simulink model "TBCC_Dyn"  (Simulink 10.0)
settings: Solver=VariableStepAuto  StartTime=0.0  StopTime=MWS.in.SimTime  FixedStep=MWS.Solve.T  RelTol=1e-3
values from neighbouring files (symbols this model uses):
  MWS = setup_Inlet(MWS)    [TBCC_setup_everything.m]
undefined symbols (not defined in the file or in its folder): combustion, diffuser, g, gama_ho, inlet_v, L_ho, nozzle, Pa, Pc_ho, R, R_ho, r_ho, stripchar_TMATS, Tc_ho, Wt_ho
libraries: Lib_Solve_ModelSource_TMATS x10, simulink_extras x7, Lib_Cntrl_FirstOrderSensor_TMATS x2, Lib_Solve_OuterLoopIntegrator_TMATS x2, Lib_Cntrl_SimplePIcontroller_TMATS x2, Lib_Turbo_Ambient_TMATS x2, Lib_Turbo_Burner_TMATS x2, Lib_Turbo_Compressor_TMATS x2, Lib_Turbo_Duct_TMATS x2, Lib_Turbo_Inlet_TMATS x2, Lib_Turbo_Nozzle_TMATS x2, Lib_Turbo_Shaft_TMATS x2
(part 1 of 2)
CloseFcn:
  | run(strcat(MWS.top_level, filesep,'GasTurbine_Dyn_Example_cleanup'))
settings Model: Creator=jwchapm2  LastModifiedBy=114-AO  SimulationMode=accelerator
settings SolverCC: AutoInsertRateTranBlk=on
settings DataIOCC: LimitDataPoints=on  SignalLoggingName=SimulationOutput
settings OptimizationCC: BlockReduction=off  DefaultParameterBehavior=Inlined  BufferReuse=off  ExpressionDepthLimit=2147483647
settings DebuggingCC: SolverPrmCheckMsg=warning  MultiTaskCondExecSysMsg=none  StateNameClashWarn=warning
settings GRTTargetCC: GeneratePreprocessorConditionals=Disable all  CombineOutputUpdateFcns=on  GRTInterface=off
settings ConfigComp: CovExternalEMLEnable=off

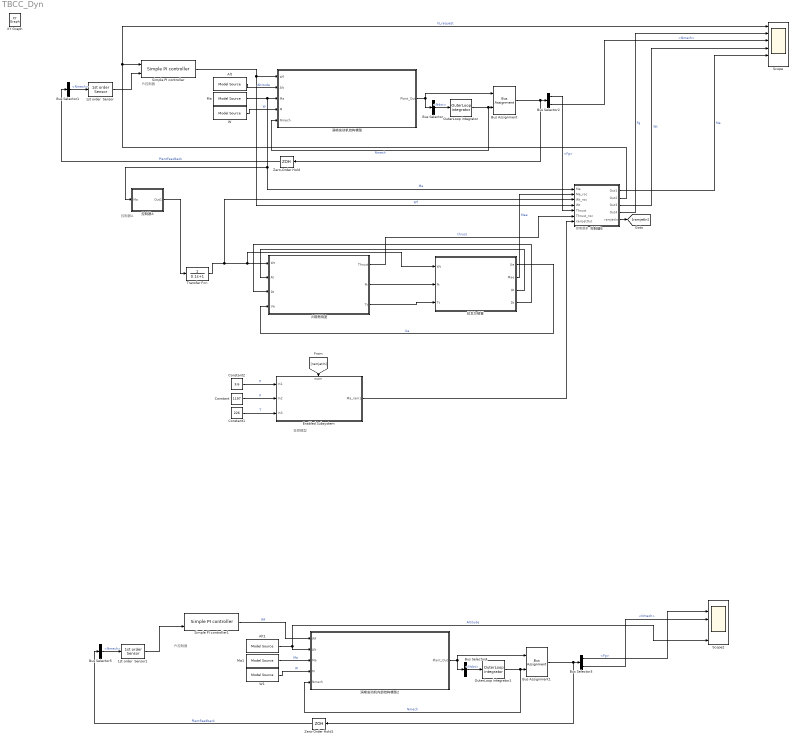
== system TBCC_Dyn ==
  note: 亚燃模型
  note: PI控制器
  note: 控制器A
  note: 控制器B
  note: PI控制器
  1st order  Sensor : Lib_Cntrl_FirstOrderSensor_TMATS/1st order  Sensor  IC_M=MWS.Solve.N_IC  Sen_Max_M=20000  Sen_Min_M=0  Gain_M=1  Tau_M=0.05  GN_EN_M=off  GN_NST_M=MWS.Solve.T  GN_C_M=1  GN_MinNoise_M=0.3  F_Gain_M=1  F_Drift_M=0
  1st order  Sensor1 : Lib_Cntrl_FirstOrderSensor_TMATS/1st order  Sensor  IC_M=MWS.Solve.N_IC  Sen_Max_M=20000  Sen_Min_M=0  Gain_M=1  Tau_M=0.05  GN_EN_M=off  GN_NST_M=MWS.Solve.T  GN_C_M=1  GN_MinNoise_M=0.3  F_Gain_M=1  F_Drift_M=0
  Alt : Lib_Solve_ModelSource_TMATS/Model Source  T_vec_M=MWS.in.t_vec  input_array_M=MWS.in.Alt
  Alt1 : Lib_Solve_ModelSource_TMATS/Model Source  T_vec_M=MWS.in.t_vec  input_array_M=MWS.in.Alt
  Bus Assignment : BusAssignment  AssignedSignals=PlantBus.Nmech
  Bus Assignment1 : BusAssignment  AssignedSignals=PlantBus.Nmech
  Bus Selector2 : BusSelector  OutputSignals=PlantBus.Fg,PlantBus.Nmech
  Bus Selector3 : BusSelector  OutputSignals=PlantBus.Fg,PlantBus.Nmech
  Bus Selector : BusSelector  OutputSignals=PlantBus.Ndot
  Bus Selector1 : BusSelector  OutputSignals=PlantBus.Nmech
  Bus Selector4 : BusSelector  OutputSignals=PlantBus.Ndot
  Bus Selector5 : BusSelector  OutputSignals=PlantBus.Nmech
  Constant : Constant  Value=1197
  Constant1 : Constant  Value=226
  Constant2 : Constant  Value=3.6
  Enabled Subsystem : Subsystem  TreatAsAtomicUnit=on
      mask Display: image('ramjet.jpg'); % Use "Edit Image" on toolstrip to change.
  Ma : Lib_Solve_ModelSource_TMATS/Model Source  T_vec_M=MWS.in.t_vec  input_array_M=MWS.in.Ma
  Ma1 : Lib_Solve_ModelSource_TMATS/Model Source  T_vec_M=MWS.in.t_vec  input_array_M=MWS.in.Ma
  OuterLoop integrator : Lib_Solve_OuterLoopIntegrator_TMATS/OuterLoop integrator  OL_IC_M=MWS.Solve.N_IC
  OuterLoop integrator1 : Lib_Solve_OuterLoopIntegrator_TMATS/OuterLoop integrator  OL_IC_M=MWS.Solve.N_IC
  Scope : Scope  NumInputPorts=6
  Scope2 : Scope  NumInputPorts=6
  Simple PI controller : Lib_Cntrl_SimplePIcontroller_TMATS/Simple PI controller  Kp_M=0.05/2  Ki_M=0.1/2  PI_IC_M=3
  Simple PI controller1 : Lib_Cntrl_SimplePIcontroller_TMATS/Simple PI controller  Kp_M=0.05/2  Ki_M=0.1/2  PI_IC_M=3
  Transfer Fcn : TransferFcn  Denominator=[0.1 1]
  W : Lib_Solve_ModelSource_TMATS/Model Source  T_vec_M=MWS.in.t_vec  input_array_M=MWS.in.W
  W1 : Lib_Solve_ModelSource_TMATS/Model Source  T_vec_M=MWS.in.t_vec  input_array_M=MWS.in.W
  Zero-Order Hold : ZeroOrderHold  SampleTime=MWS.Solve.T
  Zero-Order Hold1 : ZeroOrderHold  SampleTime=MWS.Solve.T
  拉瓦尔喷管 : Subsystem
      mask Display: image('lawaer.jpg'); % Use "Edit Image" on toolstrip to change.
  控制器A : Subsystem
  控制器B : Subsystem
  涡喷发动机内部结构模型2 : Subsystem
      mask Display: image('turbine.jpg'); % Use "Edit Image" on toolstrip to change.
  涡喷发动机结构模型 : Subsystem
      mask Display: image('turbine.jpg'); % Use "Edit Image" on toolstrip to change.
  火箭燃烧室 : Subsystem
      mask Display: image('rocket.jpg'); % Use "Edit Image" on toolstrip to change.
  XY Graph : simulink/Sinks/XY Graph  IOType=viewer  xmin=-1  xmax=1  ymin=-1  ymax=1  st=-1
  wires:
  Zero-Order Hold/1 -> Bus Selector1/1  "PlantFeedback"
  涡喷发动机结构模型/1(Plant_Out) -> Bus Selector/1, Bus Assignment/1
  Bus Selector/1 -> OuterLoop integrator/1  "<Ndot>"
  Bus Assignment/1 -> Bus Selector2/1, Zero-Order Hold/1
  OuterLoop integrator/1 -> 涡喷发动机结构模型/5(Nmech), Bus Assignment/2  "Nmech"
  Bus Selector1/1 -> 1st order  Sensor/1  "<Nmech>"
  Simple PI controller/1 -> 涡喷发动机结构模型/1(Wf), 控制器B/4(Wt)  "Wf"
  1st order  Sensor/1 -> Simple PI controller/2
  Alt/1 -> 涡喷发动机结构模型/2(Alt)  "Altitude"
  Ma/1 -> 控制器B/1(Ma), 控制器A/1(Ma), 涡喷发动机结构模型/3(Ma)  "Ma"
  W/1 -> 涡喷发动机结构模型/4(M)  "W"
  Bus Selector2/2 -> Scope/3  "<Nmech>"
  拉瓦尔喷管/4(Dt) -> 火箭燃烧室/3(Dt)
  Transfer Fcn/1 -> 控制器B/3(Wt_roc), 拉瓦尔喷管/1(Wt), 火箭燃烧室/1(Wt)
  火箭燃烧室/2(Pt) -> 拉瓦尔喷管/2(Pt)
  拉瓦尔喷管/1(Ue) -> 火箭燃烧室/4(Ue)  "Ue"
  拉瓦尔喷管/3(At) -> 火箭燃烧室/2(At)
  火箭燃烧室/3(Tt) -> 拉瓦尔喷管/3(Tt)
  拉瓦尔喷管/2(Mae) -> 控制器B/2(Ma_roc)  "Mae"
  控制器B/1(Out1) -> Scope/5  "Ma"
  控制器A/1(Out1) -> Transfer Fcn/1
  控制器B/3(Out3) -> Scope/4  "Wt"
  Bus Selector2/1 -> 控制器B/5(Thrust)  "<Fg>"
  火箭燃烧室/1(Thrust) -> 控制器B/6(Thrust_roc)  "thrust"
  控制器B/4(Out4) -> Scope/2  "Fg"
  Alt1/1 -> Scope2/6, 涡喷发动机内部结构模型2/2(Alt)  "Altitude"
  Bus Selector3/2 -> Scope2/3  "<Nmech>"
  W1/1 -> 涡喷发动机内部结构模型2/4(M)  "W"
  Ma1/1 -> 涡喷发动机内部结构模型2/3(Ma)  "Ma"
  控制器B/2(Out2) -> Simple PI controller/1, Scope/1  "N_request"
  涡喷发动机内部结构模型2/1(Plant_Out) -> Bus Selector4/1, Bus Assignment1/1
  1st order  Sensor1/1 -> Simple PI controller1/2
  Simple PI controller1/1 -> 涡喷发动机内部结构模型2/1(Wf)  "Wf"
  OuterLoop integrator1/1 -> 涡喷发动机内部结构模型2/5(Nmech), Bus Assignment1/2  "Nmech"
  Zero-Order Hold1/1 -> Bus Selector5/1  "PlantFeedback"
  Bus Assignment1/1 -> Bus Selector3/1, Zero-Order Hold1/1
  Bus Selector5/1 -> 1st order  Sensor1/1  "<Nmech>"
  Bus Selector4/1 -> OuterLoop integrator1/1  "<Ndot>"
  Bus Selector3/1 -> Scope2/2  "<Fg>"
  控制器B/5(ramjetIn) -> [ramjetIn]
  [ramjetIn] -> Enabled Subsystem/Enable
  Constant2/1 -> Enabled Subsystem/1(In1)  "P"
  Constant/1 -> Enabled Subsystem/2(In2)  "P"
  Constant1/1 -> Enabled Subsystem/3(In3)  "T"
  Enabled Subsystem/1(Ma_ram1) -> 控制器B/7(ramjetOut)

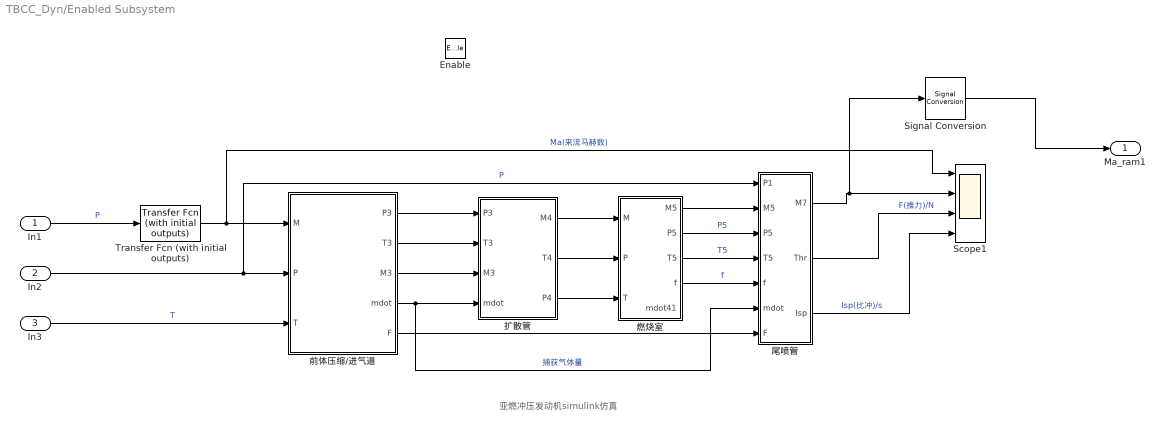
== system TBCC_Dyn/Enabled Subsystem ==
  note: 亚燃冲压发动机simulink仿真
  In1 : Inport
  In2 : Inport  Port=2
  In3 : Inport  Port=3
  Enable : EnablePort
  Scope1 : Scope  NumInputPorts=4
  Signal Conversion : SignalConversion  OverrideOpt=off
  Transfer Fcn (with initial outputs) : simulink_extras/Additional Linear/Transfer Fcn (with initial outputs)  N=[1]  D="[2  1]"  Y0=2.6  U0=0
  前体压缩/进气道 : Subsystem
  尾喷管 : Subsystem
  扩散管 : Subsystem
  燃烧室 : Subsystem
  Ma_ram1 : Outport
  wires:
  Signal Conversion/1 -> Ma_ram1/1
  扩散管/1(M4) -> 燃烧室/1(M)
  扩散管/3(P4) -> 燃烧室/3(T)
  In1/1 -> Transfer Fcn (with initial outputs)/1  "P"
  前体压缩/进气道/3(M3) -> 扩散管/3(M3)
  前体压缩/进气道/5(F) -> 尾喷管/7(F)
  前体压缩/进气道/1(P3) -> 扩散管/1(P3)
  尾喷管/1(M7) -> Signal Conversion/1, Scope1/2
  燃烧室/1(M5) -> 尾喷管/2(M5)
  In3/1 -> 前体压缩/进气道/3(T)  "T"
  燃烧室/3(T5) -> 尾喷管/4(T5)  "T5"
  In2/1 -> 尾喷管/1(P1), 前体压缩/进气道/2(P)  "P"
  Transfer Fcn (with initial outputs)/1 -> Scope1/1, 前体压缩/进气道/1(M)  "Ma(来流马赫数)"
  燃烧室/2(P5) -> 尾喷管/3(P5)  "P5"
  前体压缩/进气道/2(T3) -> 扩散管/2(T3)
  前体压缩/进气道/4(mdot) -> 尾喷管/6(mdot), 扩散管/4(mdot)  "捕获气体量"
  扩散管/2(T4) -> 燃烧室/2(P)
  尾喷管/3(Isp) -> Scope1/4  "Isp(比冲)/s"
  燃烧室/4(f) -> 尾喷管/5(f)  "f"
  尾喷管/2(Thr) -> Scope1/3  "F(推力)/N"

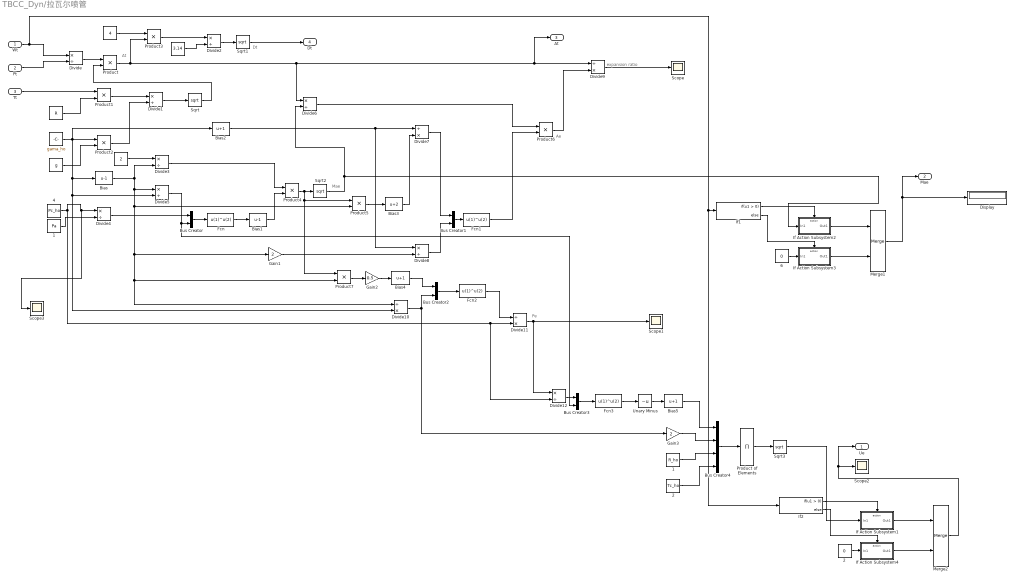
== system TBCC_Dyn/拉瓦尔喷管 ==
  note: expansion ratio
  note: Dt
  note: At
  note: Mae
  note: Ae
  note: Pe
  Wt : Inport
  Pt : Inport  Port=2
  Tt : Inport  Port=3
  " " : Constant  Value=R  SampleTime=0.6
  "  " : Constant  Value=gama_ho  SampleTime=0.6
  "   " : Constant  Value=4  SampleTime=0.6
  "    " : Constant  Value=g  SampleTime=0.6
  "     " : Constant  Value=3.14  SampleTime=0.6
  "        " : Constant  Value=2  SampleTime=0.6
  "    1" : Constant  Value=Pa  SampleTime=0.6
  "    2" : Constant  Value=0  SampleTime=0.6
  "    4" : Constant  Value=Pc_ho  SampleTime=0.6
  "    6" : Constant  Value=0  SampleTime=0.6
  " 1" : Constant  Value=R_ho  SampleTime=0.6
  " 2" : Constant  Value=Tc_ho  SampleTime=0.6
  Bias : Bias  Bias=-1
  Bias1 : Bias  Bias=-1
  Bias2 : Bias  Bias=1
  Bias3 : Bias  Bias=2
  Bias4 : Bias  Bias=1
  Bias5 : Bias  Bias=1
  Bus Creator{,1..3} (4 alike) : BusCreator  Inputs=2
  Bus Creator4 : BusCreator  Inputs=4
  Display : Display
  Divide{,1..6,8,12} (9 alike) : Product  Inputs=*/
  Divide{7,9..11} (4 alike) : Product  Inputs=/*
  Fcn{,1..3} (4 alike) : Fcn  Expr=u(1)^u(2)
  Gain1 : Gain  Gain=2
  Gain2 : Gain  Gain=0.5
  Gain3 : Gain  Gain=2
  If Action Subsystem1 : Subsystem  TreatAsAtomicUnit=on
  If Action Subsystem2 : Subsystem  TreatAsAtomicUnit=on
  If Action Subsystem3 : Subsystem  TreatAsAtomicUnit=on
  If Action Subsystem4 : Subsystem  TreatAsAtomicUnit=on
  If1 : If
  If2 : If
  Merge1 : Merge
  Merge2 : Merge
  Product{,1..7} (8 alike) : Product
  Product of Elements : Product  Inputs=*
  Scope{,1..3} (4 alike) : Scope
  Sqrt{,1..3} (4 alike) : Sqrt  SaturateOnIntegerOverflow=on
  Unary Minus : UnaryMinus
  Ue : Outport
  Mae : Outport  Port=2
  At : Outport  Port=3
  Dt : Outport  Port=4
  wires:
  Pt/1 -> Divide/2
  Divide/1 -> Product/1
  Tt/1 -> Product1/1
  " "/1 -> Product1/2
  Product1/1 -> Divide1/1
  "  "/1 -> Bias2/1, Divide10/2, Divide5/2, Bias/1, Product2/1
  "    "/1 -> Product2/2
  Product2/1 -> Divide1/2
  Divide1/1 -> Sqrt/1
  Sqrt/1 -> Product/2
  Product/1 -> Product3/2, Divide6/1, At/1, Divide9/1
  "   "/1 -> Product3/1
  Product3/1 -> Divide2/1
  "     "/1 -> Divide2/2
  Divide2/1 -> Sqrt1/1
  Sqrt1/1 -> Dt/1
  Bias/1 -> Divide10/1, Product7/2, Gain1/1, Product5/2, Divide5/1, Divide3/2
  "        "/1 -> Divide3/1
  "    1"/1 -> Divide4/2
  Divide5/1 -> Bus Creator3/2, Bus Creator/2
  Divide4/1 -> Bus Creator/1
  Bus Creator/1 -> Fcn/1
  Fcn/1 -> Bias1/1
  Divide3/1 -> Product4/1
  Bias1/1 -> Product4/2
  Product4/1 -> Product7/1, Product5/1, Sqrt2/1
  Product5/1 -> Bias3/1
  Bias3/1 -> Divide7/2
  Bias2/1 -> Divide7/1, Divide8/1
  Gain1/1 -> Divide8/2
  Divide7/1 -> Bus Creator1/1
  Divide8/1 -> Bus Creator1/2
  Bus Creator1/1 -> Fcn1/1
  Divide6/1 -> Product6/1
  Fcn1/1 -> Product6/2
  Product6/1 -> Divide9/2
  Divide9/1 -> Scope/1
  Product7/1 -> Gain2/1
  Gain2/1 -> Bias4/1
  Bias4/1 -> Bus Creator2/1
  Divide10/1 -> Gain3/1, Bus Creator2/2
  Bus Creator2/1 -> Fcn2/1
  Fcn2/1 -> Divide11/1
  Divide11/1 -> Divide12/1, Scope1/1
  Bus Creator3/1 -> Fcn3/1
  Divide12/1 -> Bus Creator3/1
  Fcn3/1 -> Unary Minus/1
  Unary Minus/1 -> Bias5/1
  Gain3/1 -> Bus Creator4/2
  " 1"/1 -> Bus Creator4/3
  " 2"/1 -> Bus Creator4/4
  Product of Elements/1 -> Sqrt3/1
  Bias5/1 -> Bus Creator4/1
  Bus Creator4/1 -> Product of Elements/1
  Merge2/1 -> Ue/1, Scope2/1
  Wt/1 -> If2/1, If1/1, Divide/1
  "    4"/1 -> Divide12/2, Divide11/2, Scope3/1, Divide4/1
  If1/2 -> If Action Subsystem3/Action
  Sqrt2/1 -> If Action Subsystem2/1(In1), Divide6/2
  "    6"/1 -> If Action Subsystem3/1(In1)
  If Action Subsystem3/1(Out1) -> Merge1/2
  If1/1 -> If Action Subsystem2/Action
  Merge1/1 -> Display/1, Mae/1
  If Action Subsystem2/1(Out1) -> Merge1/1
  If2/2 -> If Action Subsystem4/Action
  If2/1 -> If Action Subsystem1/Action
  "    2"/1 -> If Action Subsystem4/1(In1)
  If Action Subsystem4/1(Out1) -> Merge2/2
  If Action Subsystem1/1(Out1) -> Merge2/1
  Sqrt3/1 -> If Action Subsystem1/1(In1)

== system TBCC_Dyn/控制器A ==
  Ma : Inport
  "    3" : Constant  Value=0  SampleTime=0.6
  If : If  IfExpression=u1 >= 1
  If Action Subsystem : Subsystem  TreatAsAtomicUnit=on
  If Action Subsystem1 : Subsystem  TreatAsAtomicUnit=on
  Merge : Merge
  Wt : Constant  Value=Wt_ho  SampleTime=0.6
  Out1 : Outport
  wires:
  Merge/1 -> Out1/1
  "    3"/1 -> If Action Subsystem1/1(In1)
  Wt/1 -> If Action Subsystem/1(In1)
  If/2 -> If Action Subsystem1/Action
  If Action Subsystem/1(Out1) -> Merge/1
  If/1 -> If Action Subsystem/Action
  If Action Subsystem1/1(Out1) -> Merge/2
  Ma/1 -> If/1

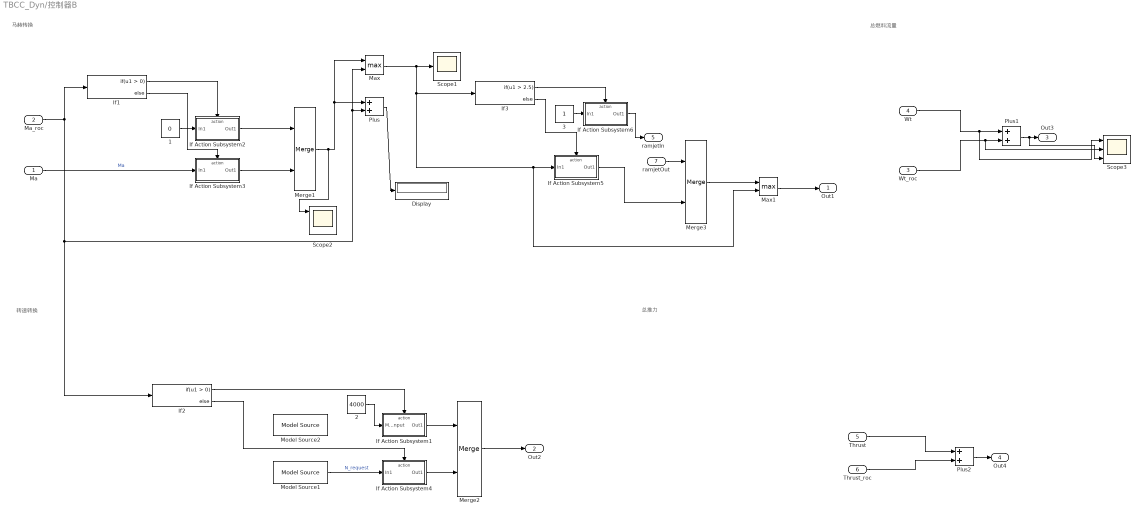
== system TBCC_Dyn/控制器B ==
  note: 总燃料流量
  note: 马赫转换
  note: 转速转换
  note: 总推力
  Ma : Inport
  Ma_roc : Inport  Port=2
  Wt_roc : Inport  Port=3
  Wt : Inport  Port=4
  Thrust : Inport  Port=5
  Thrust_roc : Inport  Port=6
  ramjetOut : Inport  Port=7
  "    1" : Constant  Value=0  SampleTime=0.6
  "    2" : Constant  Value=4000  SampleTime=0.6
  "    3" : Constant  SampleTime=0.6
  Display : Display
  If Action Subsystem1 : Subsystem  TreatAsAtomicUnit=on
  If Action Subsystem2 : Subsystem  TreatAsAtomicUnit=on
  If Action Subsystem3 : Subsystem  TreatAsAtomicUnit=on
  If Action Subsystem4 : Subsystem  TreatAsAtomicUnit=on
  If Action Subsystem5 : Subsystem  TreatAsAtomicUnit=on
  If Action Subsystem6 : Subsystem  TreatAsAtomicUnit=on
  If1 : If
  If2 : If
  If3 : If  IfExpression=u1 > 2.5
  Max : MinMax  Function=max  Inputs=2
  Max1 : MinMax  Function=max  Inputs=2
  Merge1 : Merge  InitialOutput=[1]
  Merge2 : Merge  InitialOutput=[1]
  Merge3 : Merge  InitialOutput=[1]
  Model Source1 : Lib_Solve_ModelSource_TMATS/Model Source  T_vec_M=MWS.in.t_vec  input_array_M=MWS.in.Ndmd
  Model Source2 : Lib_Solve_ModelSource_TMATS/Model Source  T_vec_M=MWS.in.t_vec  input_array_M=MWS.in.Ndmd_stop
  Plus : Sum
  Plus1 : Sum
  Plus2 : Sum
  Scope1 : Scope  NumInputPorts=3
  Scope2 : Scope  NumInputPorts=3
  Scope3 : Scope  NumInputPorts=3
  Out1 : Outport
  Out2 : Outport  Port=2
  Out3 : Outport  Port=3
  Out4 : Outport  Port=4
  ramjetIn : Outport  Port=5
  wires:
  If1/1 -> If Action Subsystem2/Action
  "    1"/1 -> If Action Subsystem2/1(In1)
  Merge1/1 -> Scope2/1, Max/1, Plus/1
  If Action Subsystem3/1(Out1) -> Merge1/2
  Plus/1 -> Display/1
  Ma_roc/1 -> If1/1, If2/1, Max/2, Plus/2
  Ma/1 -> If Action Subsystem3/1(In1)  "Ma"
  If1/2 -> If Action Subsystem3/Action
  If Action Subsystem2/1(Out1) -> Merge1/1
  Max/1 -> Max1/2, If Action Subsystem5/1(In1), If3/1, Scope1/2
  Model Source1/1 -> If Action Subsystem4/1(In1)  "N_request"
  If Action Subsystem1/1(Out1) -> Merge2/1
  If Action Subsystem4/1(Out1) -> Merge2/2
  If2/2 -> If Action Subsystem4/Action
  Wt/1 -> Scope3/1, Plus1/1
  Wt_roc/1 -> Scope3/2, Plus1/2
  Plus1/1 -> Scope3/3, Out3/1
  Merge2/1 -> Out2/1
  Thrust/1 -> Plus2/1
  Thrust_roc/1 -> Plus2/2
  Plus2/1 -> Out4/1
  If2/1 -> If Action Subsystem1/Action
  "    2"/1 -> If Action Subsystem1/1(Model_Input)
  If3/2 -> If Action Subsystem5/Action
  If Action Subsystem5/1(Out1) -> Merge3/2
  Merge3/1 -> Max1/1
  If3/1 -> If Action Subsystem6/Action
  If Action Subsystem6/1(Out1) -> ramjetIn/1
  "    3"/1 -> If Action Subsystem6/1(In1)
  ramjetOut/1 -> Merge3/1
  Max1/1 -> Out1/1

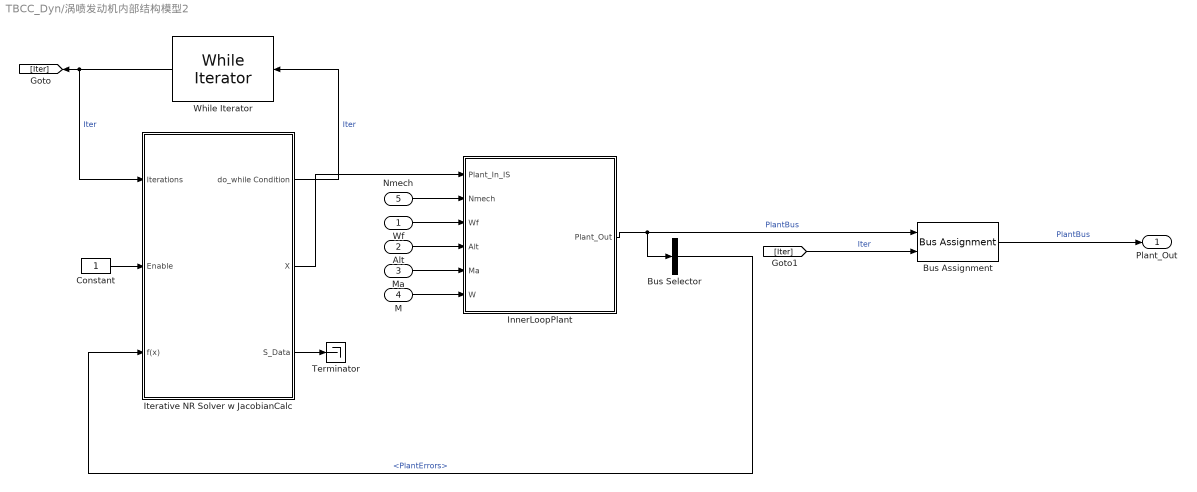
== system TBCC_Dyn/涡喷发动机内部结构模型2 ==
  Wf : Inport
  Alt : Inport  Port=2
  Ma : Inport  Port=3
  M : Inport  Port=4
  Nmech : Inport  Port=5
  Bus Assignment : BusAssignment  AssignedSignals=PlantBus.Iter
  Bus Selector : BusSelector  OutputSignals=PlantErrors
  Constant : Constant
  InnerLoopPlant : Subsystem
  Iterative NR Solver w JacobianCalc : Subsystem  AncestorBlock=Lib_Solve_IterNRSolverJC_TMATS/Iterative NR Solver w JacobianCalc  mask(T-MATS: Iterative NR Solver w Jacobian Calc Library Block){SJac_Per_M=MWS.Solve.J_Calc_Per, SNR_IC_M=MWS.Solve.NR_IC, SNR_DX_M=MWS.Solve.NR_dx, SNR_Mx_M=100000, SNR_Mn_M=0.0001, SJacobianAttempts_M=MWS.Solve.NR_Jac_Re, Cond_Limits_M=MWS.Solve.C_Lim}
      mask prompts: SJac_Per_M "SJac_Per_M - Jacobian Perturbation size (frac) (nxm)"; SNR_IC_M "SNR_IC_M - Newton Raphson Initial Conditions (mx1)"; SNR_DX_M "SNR_DX_M - Newton Raphson step size limiter (%) (1x1)"; SNR_Mx_M "SNR_Mx_M - Newton Raphson max limit (1x1 or mx1)"; SNR_Mn_M "SNR_Mn_M - Newton Raphson min limit (1x1 or mx1)"; SJacobianAttempts_M "SJacobianAttempts_M - Newton Raphson attempts before the Jacobian recalculation (1x1)"; Cond_Limits_M "Cond_Limits_M - Iteration Conditions Limits (mx1 or 1x1)"
      mask help:
      | The Iterative Newton Raphson Solver with Jacobian Calculator block will
      | supply the inputs to iteratively drive the outputs of a system to zero.
      |
      | This will be performed in three steps.
      | 1) Jabobian calculator sends Perturbations to the plant then calculates the plant
      | Jacboian based on the system response
      | 2) The Newton Raphson will use the inverse of the Jacobian to iteratively step the
      | system toward solution.
      | 3) Once the solution has satisfied the conditions the Newton Raphson is shut off.
      |
      | This module is designed for dynamic systems and should be paired with
      | a "do... while" block in Simulink. The "do...while" block and this module
      | should both be located in the same subsystem as the plant that is to be solved for.
      mask init:
      | if isequal(size(SNR_Mx_M),size(SNR_IC_M))
      | elseif isequal(size(SNR_Mx_M),[1 1])
      | else
      |     disp('NR_Mx_Lim_M must be the same size as NR_IC_M or a constant')
      | end
      | 
      | if isequal(size(SNR_Mn_M),size(SNR_IC_M))
      | elseif isequal(size(SNR_Mn_M),[1 1])
      | else
      |     disp('NR_Mn_Lim_M must be the same size as NR_IC_M or a constant')
      | end
      mask Help: web(which('Solver_TMATS_INRSwJC.html'),'-helpbrowser')
  Terminator : Terminator
  While Iterator : WhileIterator  MaxIters=MWS.Solve.Max_Iter  WhileBlockType=do-while  ShowIterationPort=on
  Plant_Out : Outport
  wires:
  Bus Selector/1 -> Iterative NR Solver w JacobianCalc/3(f(x))  "<PlantErrors>"
  While Iterator/1 -> [Iter], Iterative NR Solver w JacobianCalc/1(Iterations)  "Iter"
  InnerLoopPlant/1(Plant_Out) -> Bus Assignment/1, Bus Selector/1  "PlantBus"
  Iterative NR Solver w JacobianCalc/2(X) -> InnerLoopPlant/1(Plant_In_IS)
  Iterative NR Solver w JacobianCalc/1(do_while Condition) -> While Iterator/1  "Iter"
  Iterative NR Solver w JacobianCalc/3(S_Data) -> Terminator/1
  Constant/1 -> Iterative NR Solver w JacobianCalc/2(Enable)
  [Iter] -> Bus Assignment/2  "Iter"
  Bus Assignment/1 -> Plant_Out/1  "PlantBus"
  Nmech/1 -> InnerLoopPlant/2(Nmech)
  Wf/1 -> InnerLoopPlant/3(Wf)
  Alt/1 -> InnerLoopPlant/4(Alt)
  Ma/1 -> InnerLoopPlant/5(Ma)
  M/1 -> InnerLoopPlant/6(W)

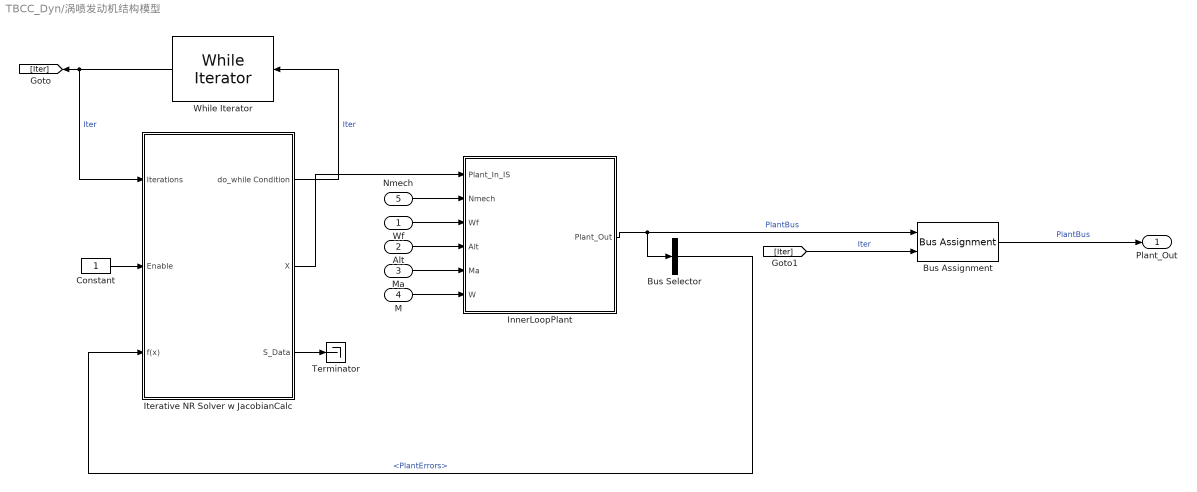
== system TBCC_Dyn/涡喷发动机结构模型 ==
  Wf : Inport
  Alt : Inport  Port=2
  Ma : Inport  Port=3
  M : Inport  Port=4
  Nmech : Inport  Port=5
  Bus Assignment : BusAssignment  AssignedSignals=PlantBus.Iter
  Bus Selector : BusSelector  OutputSignals=PlantErrors
  Constant : Constant
  InnerLoopPlant : Subsystem
  Iterative NR Solver w JacobianCalc : Subsystem  AncestorBlock=Lib_Solve_IterNRSolverJC_TMATS/Iterative NR Solver w JacobianCalc  mask(T-MATS: Iterative NR Solver w Jacobian Calc Library Block){SJac_Per_M=MWS.Solve.J_Calc_Per, SNR_IC_M=MWS.Solve.NR_IC, SNR_DX_M=MWS.Solve.NR_dx, SNR_Mx_M=100000, SNR_Mn_M=0.0001, SJacobianAttempts_M=MWS.Solve.NR_Jac_Re, Cond_Limits_M=MWS.Solve.C_Lim}
      mask prompts: SJac_Per_M "SJac_Per_M - Jacobian Perturbation size (frac) (nxm)"; SNR_IC_M "SNR_IC_M - Newton Raphson Initial Conditions (mx1)"; SNR_DX_M "SNR_DX_M - Newton Raphson step size limiter (%) (1x1)"; SNR_Mx_M "SNR_Mx_M - Newton Raphson max limit (1x1 or mx1)"; SNR_Mn_M "SNR_Mn_M - Newton Raphson min limit (1x1 or mx1)"; SJacobianAttempts_M "SJacobianAttempts_M - Newton Raphson attempts before the Jacobian recalculation (1x1)"; Cond_Limits_M "Cond_Limits_M - Iteration Conditions Limits (mx1 or 1x1)"
      mask help:
      | The Iterative Newton Raphson Solver with Jacobian Calculator block will
      | supply the inputs to iteratively drive the outputs of a system to zero.
      |
      | This will be performed in three steps.
      | 1) Jabobian calculator sends Perturbations to the plant then calculates the plant
      | Jacboian based on the system response
      | 2) The Newton Raphson will use the inverse of the Jacobian to iteratively step the
      | system toward solution.
      | 3) Once the solution has satisfied the conditions the Newton Raphson is shut off.
      |
      | This module is designed for dynamic systems and should be paired with
      | a "do... while" block in Simulink. The "do...while" block and this module
      | should both be located in the same subsystem as the plant that is to be solved for.
      mask init: same as TBCC_Dyn/涡喷发动机内部结构模型2/Iterative NR Solver w JacobianCalc
      mask Help: web(which('Solver_TMATS_INRSwJC.html'),'-helpbrowser')
  Terminator : Terminator
  While Iterator : WhileIterator  MaxIters=MWS.Solve.Max_Iter  WhileBlockType=do-while  ShowIterationPort=on
  Plant_Out : Outport
  wires:
  Bus Selector/1 -> Iterative NR Solver w JacobianCalc/3(f(x))  "<PlantErrors>"
  While Iterator/1 -> [Iter], Iterative NR Solver w JacobianCalc/1(Iterations)  "Iter"
  InnerLoopPlant/1(Plant_Out) -> Bus Assignment/1, Bus Selector/1  "PlantBus"
  Iterative NR Solver w JacobianCalc/2(X) -> InnerLoopPlant/1(Plant_In_IS)
  Iterative NR Solver w JacobianCalc/1(do_while Condition) -> While Iterator/1  "Iter"
  Iterative NR Solver w JacobianCalc/3(S_Data) -> Terminator/1
  Constant/1 -> Iterative NR Solver w JacobianCalc/2(Enable)
  [Iter] -> Bus Assignment/2  "Iter"
  Bus Assignment/1 -> Plant_Out/1  "PlantBus"
  Nmech/1 -> InnerLoopPlant/2(Nmech)
  Wf/1 -> InnerLoopPlant/3(Wf)
  Alt/1 -> InnerLoopPlant/4(Alt)
  Ma/1 -> InnerLoopPlant/5(Ma)
  M/1 -> InnerLoopPlant/6(W)

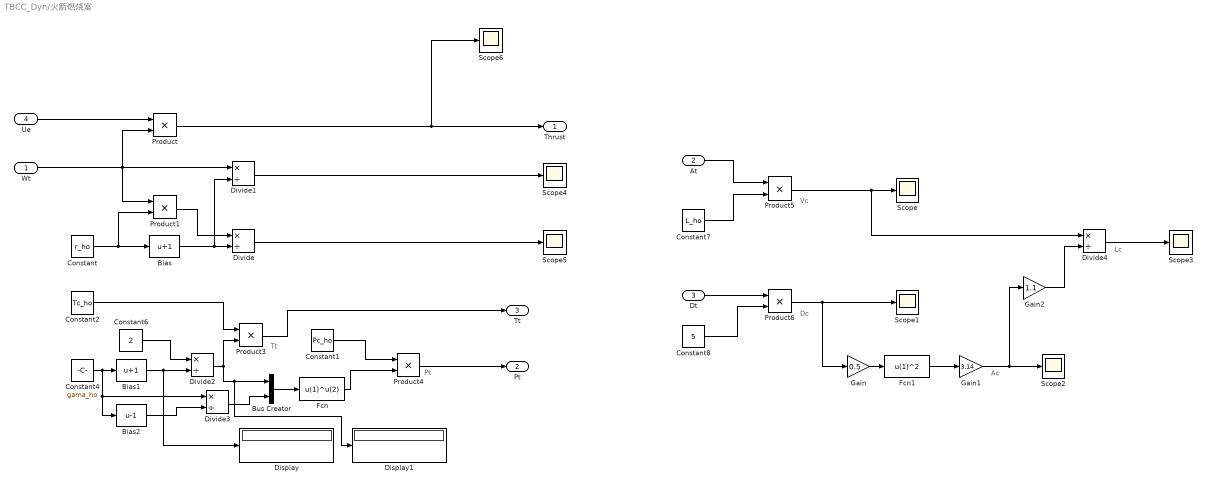
== system TBCC_Dyn/火箭燃烧室 ==
  note: Vc
  note: Tt
  note: Pt
  note: Dc
  note: Ac
  note: Lc
  Wt : Inport
  At : Inport  Port=2
  Dt : Inport  Port=3
  Ue : Inport  Port=4
  Bias : Bias  Bias=1
  Bias1 : Bias  Bias=1
  Bias2 : Bias  Bias=-1
  Bus Creator : BusCreator  Inputs=2
  Constant : Constant  Value=r_ho  SampleTime=0.6
  Constant1 : Constant  Value=Pc_ho  SampleTime=0.6
  Constant2 : Constant  Value=Tc_ho  SampleTime=0.6
  Constant4 : Constant  Value=gama_ho  SampleTime=0.6
  Constant6 : Constant  Value=2  SampleTime=0.6
  Constant7 : Constant  Value=L_ho  SampleTime=0.6
  Constant8 : Constant  Value=5  SampleTime=0.6
  Display : Display
      settings: Decimation=2
  Display1 : Display
      settings: Decimation=2
  Divide{,1..4} (5 alike) : Product  Inputs=*/
  Fcn : Fcn  Expr=u(1)^u(2)
  Fcn1 : Fcn  Expr=u(1)^2
  Gain : Gain  Gain=0.5
  Gain1 : Gain  Gain=3.14
  Gain2 : Gain  Gain=1.1
  Product{,1,3..6} (6 alike) : Product
  Scope{,1..6} (7 alike) : Scope
  Thrust : Outport
  Pt : Outport  Port=2
  Tt : Outport  Port=3
  wires:
  Wt/1 -> Product/2, Product1/1, Divide1/1
  Ue/1 -> Product/1
  Constant/1 -> Product1/2, Bias/1
  Bias/1 -> Divide/2, Divide1/2
  Product1/1 -> Divide/1
  Product/1 -> Scope6/1, Thrust/1
  Divide1/1 -> Scope4/1
  Divide/1 -> Scope5/1
  Constant4/1 -> Bias2/1, Divide3/1, Bias1/1
  Constant6/1 -> Divide2/1
  Bias1/1 -> Display/1, Divide2/2
  Constant2/1 -> Product3/1
  Divide2/1 -> Product3/2, Display1/1, Bus Creator/1
  Bias2/1 -> Divide3/2
  Divide3/1 -> Bus Creator/2
  Bus Creator/1 -> Fcn/1
  Fcn/1 -> Product4/2
  Constant1/1 -> Product4/1
  Product4/1 -> Pt/1
  Product3/1 -> Tt/1
  At/1 -> Product5/1
  Constant7/1 -> Product5/2
  Product5/1 -> Divide4/1, Scope/1
  Dt/1 -> Product6/1
  Constant8/1 -> Product6/2
  Product6/1 -> Gain/1, Scope1/1
  Gain/1 -> Fcn1/1
  Fcn1/1 -> Gain1/1
  Gain1/1 -> Gain2/1, Scope2/1
  Gain2/1 -> Divide4/2
  Divide4/1 -> Scope3/1

== system TBCC_Dyn/Enabled Subsystem/前体压缩/进气道 ==
  M : Inport
  P : Inport  Port=2
  T : Inport  Port=3
  Demux : Demux  Outputs=5
  Interpreted MATLAB Function1 : MATLABFcn  MATLABFcn=inlet_v(u(1),u(2),u(3))  OutputDimensions=5
  Mux3 : Mux  Inputs=3
  P3 : Outport
  T3 : Outport  Port=2
  M3 : Outport  Port=3
  mdot : Outport  Port=4
  F : Outport  Port=5
  wires:
  Mux3/1 -> Interpreted MATLAB Function1/1
  Demux/1 -> mdot/1  "mdot"
  Interpreted MATLAB Function1/1 -> Demux/1
  M/1 -> Mux3/1
  P/1 -> Mux3/2
  Demux/5 -> F/1  "F"
  T/1 -> Mux3/3
  Demux/2 -> P3/1  "P3"
  Demux/3 -> T3/1  "T3"
  Demux/4 -> M3/1  "M3"

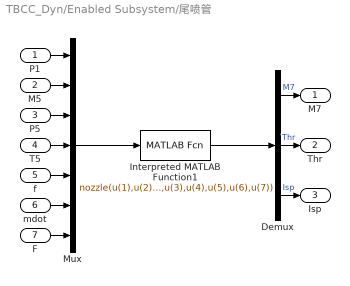
== system TBCC_Dyn/Enabled Subsystem/尾喷管 ==
  P1 : Inport
  M5 : Inport  Port=2
  P5 : Inport  Port=3
  T5 : Inport  Port=4
  f : Inport  Port=5
  mdot : Inport  Port=6
  F : Inport  Port=7
  Demux : Demux  Outputs=3
  Interpreted MATLAB Function1 : MATLABFcn  MATLABFcn=nozzle(u(1),u(2),u(3),u(4),u(5),u(6),u(7))  OutputDimensions=3
  Mux : Mux  Inputs=7
  M7 : Outport
  Thr : Outport  Port=2
  Isp : Outport  Port=3
  wires:
  Demux/3 -> Isp/1  "Isp"
  f/1 -> Mux/5
  mdot/1 -> Mux/6
  Interpreted MATLAB Function1/1 -> Demux/1
  Mux/1 -> Interpreted MATLAB Function1/1
  P5/1 -> Mux/3
  Demux/1 -> M7/1  "M7"
  F/1 -> Mux/7
  Demux/2 -> Thr/1  "Thr"
  M5/1 -> Mux/2
  P1/1 -> Mux/1
  T5/1 -> Mux/4

== system TBCC_Dyn/Enabled Subsystem/扩散管 ==
  P3 : Inport
  T3 : Inport  Port=2
  M3 : Inport  Port=3
  mdot : Inport  Port=4
  Demux : Demux  Outputs=3
  Interpreted MATLAB Function1 : MATLABFcn  MATLABFcn=diffuser(u(1),u(2),u(3),u(4))  OutputDimensions=3
  Mux3 : Mux
  M4 : Outport
  T4 : Outport  Port=2
  P4 : Outport  Port=3
  wires:
  Demux/3 -> P4/1  "P4"
  T3/1 -> Mux3/2
  M3/1 -> Mux3/3
  Demux/2 -> T4/1  "T4"
  Interpreted MATLAB Function1/1 -> Demux/1
  Mux3/1 -> Interpreted MATLAB Function1/1
  mdot/1 -> Mux3/4
  P3/1 -> Mux3/1
  Demux/1 -> M4/1  "M4"

== system TBCC_Dyn/Enabled Subsystem/燃烧室 ==
  M : Inport
  P : Inport  Port=2
  T : Inport  Port=3
  Demux : Demux  Outputs=5
  Interpreted MATLAB Function1 : MATLABFcn  MATLABFcn=combustion(u(1),u(2),u(3))  OutputDimensions=5
  Mux : Mux  Inputs=3
  M5 : Outport
  P5 : Outport  Port=2
  T5 : Outport  Port=3
  f : Outport  Port=4
  mdot41 : Outport  Port=5
  wires:
  Mux/1 -> Interpreted MATLAB Function1/1
  Demux/4 -> f/1
  M/1 -> Mux/1
  P/1 -> Mux/2
  Demux/3 -> T5/1
  Interpreted MATLAB Function1/1 -> Demux/1
  Demux/5 -> mdot41/1
  Demux/2 -> P5/1
  Demux/1 -> M5/1
  T/1 -> Mux/3

== system TBCC_Dyn/拉瓦尔喷管/If Action Subsystem1 ==
  In1 : Inport
  Action Port : ActionPort  ActionPortLabel=if(u1 > 0)
  Transfer Fcn1 : TransferFcn  Denominator=[1 1]
  Out1 : Outport
  wires:
  In1/1 -> Transfer Fcn1/1
  Transfer Fcn1/1 -> Out1/1

== system TBCC_Dyn/拉瓦尔喷管/If Action Subsystem2 ==
  In1 : Inport
  Action Port : ActionPort  ActionPortLabel=if(u1 > 0)
  Transfer Fcn2 : TransferFcn  Denominator=[5 1]
  Out1 : Outport
  wires:
  In1/1 -> Transfer Fcn2/1
  Transfer Fcn2/1 -> Out1/1

== system TBCC_Dyn/拉瓦尔喷管/If Action Subsystem3 ==
  In1 : Inport
  Action Port : ActionPort  ActionPortLabel=else
  Out1 : Outport
  wires:
  In1/1 -> Out1/1

== system TBCC_Dyn/拉瓦尔喷管/If Action Subsystem4 ==
  In1 : Inport
  Action Port : ActionPort  ActionPortLabel=else
  Out1 : Outport
  wires:
  In1/1 -> Out1/1

== system TBCC_Dyn/控制器A/If Action Subsystem ==
  In1 : Inport
  Action Port : ActionPort  ActionPortLabel=if(u1 >= 1)
  Transport Delay : TransportDelay  DelayTime=0
  Out1 : Outport
  wires:
  In1/1 -> Transport Delay/1
  Transport Delay/1 -> Out1/1

== system TBCC_Dyn/控制器A/If Action Subsystem1 ==
  In1 : Inport
  Action Port : ActionPort  ActionPortLabel=else
  Out1 : Outport
  wires:
  In1/1 -> Out1/1

== system TBCC_Dyn/控制器B/If Action Subsystem1 ==
  Model_Input : Inport
  Action Port : ActionPort  ActionPortLabel=if(u1 > 0)
  Display : Display
  If Action Subsystem1 : Subsystem  TreatAsAtomicUnit=on
  If Action Subsystem2 : Subsystem  TreatAsAtomicUnit=on
  If3 : If  IfExpression=u1 <= 0
  Merge2 : Merge  InitialOutput=[1]
  Model Source1 : Lib_Solve_ModelSource_TMATS/Model Source  T_vec_M=MWS.in.t_vec  input_array_M=MWS.in.Ndmd_stop1
  Scope : Scope
  Transfer Fcn (with initial outputs) : simulink_extras/Additional Linear/Transfer Fcn (with initial outputs)  N=[1]  D="[10  1]"  Y0=11000  U0=0
  Transport Delay : TransportDelay  DelayTime=0.4  InitialOutput=11000
  Out1 : Outport
  wires:
  If3/2 -> If Action Subsystem2/Action
  If Action Subsystem2/1(Out1) -> Merge2/2
  If3/1 -> If Action Subsystem1/Action
  Model Source1/1 -> If Action Subsystem1/1(In1)
  If Action Subsystem1/1(Out1) -> Merge2/1
  Merge2/1 -> Out1/1
  Model_Input/1 -> Transport Delay/1
  Transfer Fcn (with initial outputs)/1 -> Scope/1, Display/1, If3/1
  Transport Delay/1 -> Transfer Fcn (with initial outputs)/1, If Action Subsystem2/1(In1)

== system TBCC_Dyn/控制器B/If Action Subsystem2 ==
  note: 惯性环节
  In1 : Inport
  Action Port : ActionPort  ActionPortLabel=if(u1 > 0)
  Transfer Fcn (with initial outputs) : simulink_extras/Additional Linear/Transfer Fcn (with initial outputs)  N=[1]  D="[2  1]"  Y0=1  U0=0
  Transport Delay : TransportDelay  DelayTime=5  InitialOutput=1
  Out1 : Outport
  wires:
  Transfer Fcn (with initial outputs)/1 -> Out1/1
  Transport Delay/1 -> Transfer Fcn (with initial outputs)/1
  In1/1 -> Transport Delay/1

== system TBCC_Dyn/控制器B/If Action Subsystem3 ==
  In1 : Inport
  Action Port : ActionPort  ActionPortLabel=else
  Out1 : Outport
  wires:
  In1/1 -> Out1/1

== system TBCC_Dyn/控制器B/If Action Subsystem4 ==
  In1 : Inport
  Action Port : ActionPort  ActionPortLabel=else
  Out1 : Outport
  wires:
  In1/1 -> Out1/1

== system TBCC_Dyn/控制器B/If Action Subsystem5 ==
  In1 : Inport
  Action Port : ActionPort  ActionPortLabel=else
  Out1 : Outport
  wires:
  In1/1 -> Out1/1

== system TBCC_Dyn/控制器B/If Action Subsystem6 ==
  In1 : Inport
  Action Port : ActionPort  ActionPortLabel=if(u1 > 2.5)
  Transport Delay : TransportDelay  DelayTime=10
  Out1 : Outport
  wires:
  In1/1 -> Transport Delay/1
  Transport Delay/1 -> Out1/1

== system TBCC_Dyn/涡喷发动机内部结构模型2/InnerLoopPlant ==
  Plant_In_IS : Inport
  Nmech : Inport  Port=2
  Wf : Inport  Port=3
  Alt : Inport  Port=4
  Ma : Inport  Port=5
  W : Inport  Port=6
  Bus Creator : BusCreator  Inputs=2
  Demux1 : Demux  Outputs=3
  Engine : Subsystem
  Plant_Out : Outport
  wires:
  Engine/1(PlantBus) -> Bus Creator/1  "PlantBus"
  Engine/2(NormFlowErrorsOut) -> Bus Creator/2  "PlantErrors"
  Bus Creator/1 -> Plant_Out/1
  Demux1/2 -> Engine/2(Rline)
  Demux1/3 -> Engine/3(PR)
  Plant_In_IS/1 -> Demux1/1
  Nmech/1 -> Engine/4(Nmech)
  Wf/1 -> Engine/5(Wf)
  Alt/1 -> Engine/6(Alt)
  Ma/1 -> Engine/7(Ma)
  W/1 -> Engine/1(W)

== system TBCC_Dyn/涡喷发动机内部结构模型2/Iterative NR Solver w JacobianCalc ==
  Iterations : Inport  PortDimensions=1
  Enable : Inport  Port=2  PortDimensions=1
  f(x) : Inport  Port=3  PortDimensions=length(SNR_IC_M)
  Bus Creator : BusCreator  Inputs=2
  JC w Reset : Subsystem
  Logical Operator : Logic  AllPortsSameDT=off  OutDataTypeStr=boolean
  NRwCond : Subsystem
  do_while Condition : Outport  PortDimensions=1
  X : Outport  Port=2  PortDimensions=length(SNR_IC_M)
  S_Data : Outport  Port=3
  wires:
  JC w Reset/2(JacFailed) -> Bus Creator/2
  Bus Creator/1 -> S_Data/1
  Logical Operator/1 -> do_while Condition/1
  Enable/1 -> Logical Operator/1, NRwCond/Enable, JC w Reset/Enable
  JC w Reset/5(inv(J)) -> NRwCond/3(inv(f'(x)))
  JC w Reset/4(JC_Active) -> NRwCond/2(JC_Active)
  JC w Reset/3(X_out) -> X/1
  JC w Reset/1(J) -> Bus Creator/1
  NRwCond/2(x(n+1)) -> JC w Reset/3(x(n+1))
  Iterations/1 -> JC w Reset/2(Iter)
  NRwCond/1(CCnd) -> Logical Operator/2
  f(x)/1 -> JC w Reset/1(f(x)), NRwCond/1(f(x))

== system TBCC_Dyn/涡喷发动机结构模型/InnerLoopPlant ==
  Plant_In_IS : Inport
  Nmech : Inport  Port=2
  Wf : Inport  Port=3
  Alt : Inport  Port=4
  Ma : Inport  Port=5
  W : Inport  Port=6
  Bus Creator : BusCreator  Inputs=2
  Demux1 : Demux  Outputs=3
  Engine : Subsystem
  Plant_Out : Outport
  wires:
  Engine/1(PlantBus) -> Bus Creator/1  "PlantBus"
  Engine/2(NormFlowErrorsOut) -> Bus Creator/2  "PlantErrors"
  Bus Creator/1 -> Plant_Out/1
  Demux1/2 -> Engine/2(Rline)
  Demux1/3 -> Engine/3(PR)
  Plant_In_IS/1 -> Demux1/1
  Nmech/1 -> Engine/4(Nmech)
  Wf/1 -> Engine/5(Wf)
  Alt/1 -> Engine/6(Alt)
  Ma/1 -> Engine/7(Ma)
  W/1 -> Engine/1(W)

== system TBCC_Dyn/涡喷发动机结构模型/Iterative NR Solver w JacobianCalc ==
  Iterations : Inport  PortDimensions=1
  Enable : Inport  Port=2  PortDimensions=1
  f(x) : Inport  Port=3  PortDimensions=length(SNR_IC_M)
  Bus Creator : BusCreator  Inputs=2
  JC w Reset : Subsystem
  Logical Operator : Logic  AllPortsSameDT=off  OutDataTypeStr=boolean
  NRwCond : Subsystem
  do_while Condition : Outport  PortDimensions=1
  X : Outport  Port=2  PortDimensions=length(SNR_IC_M)
  S_Data : Outport  Port=3
  wires:
  JC w Reset/2(JacFailed) -> Bus Creator/2
  Bus Creator/1 -> S_Data/1
  Logical Operator/1 -> do_while Condition/1
  Enable/1 -> Logical Operator/1, NRwCond/Enable, JC w Reset/Enable
  JC w Reset/5(inv(J)) -> NRwCond/3(inv(f'(x)))
  JC w Reset/4(JC_Active) -> NRwCond/2(JC_Active)
  JC w Reset/3(X_out) -> X/1
  JC w Reset/1(J) -> Bus Creator/1
  NRwCond/2(x(n+1)) -> JC w Reset/3(x(n+1))
  Iterations/1 -> JC w Reset/2(Iter)
  NRwCond/1(CCnd) -> Logical Operator/2
  f(x)/1 -> JC w Reset/1(f(x)), NRwCond/1(f(x))

== system TBCC_Dyn/控制器B/If Action Subsystem1/If Action Subsystem1 ==
  In1 : Inport
  Action Port : ActionPort  ActionPortLabel=if(u1 <= 0)
  If Action Subsystem1 : Subsystem  TreatAsAtomicUnit=on
  If Action Subsystem2 : Subsystem  TreatAsAtomicUnit=on
  If3 : If  IfExpression=u1 <= 1
  Merge : Merge
  Model Source2 : Lib_Solve_ModelSource_TMATS/Model Source  T_vec_M=MWS.in.t_vec  input_array_M=MWS.in.Ndmd_stop2
  Transfer Fcn (with initial outputs) : simulink_extras/Additional Linear/Transfer Fcn (with initial outputs)  N=[1]  D="[10  1]"  Y0=7020  U0=0
  Out1 : Outport
  wires:
  Transfer Fcn (with initial outputs)/1 -> If3/1
  If3/1 -> If Action Subsystem1/Action
  If3/2 -> If Action Subsystem2/Action
  In1/1 -> If Action Subsystem2/1(In1), Transfer Fcn (with initial outputs)/1
  Model Source2/1 -> If Action Subsystem1/1(In1)
  If Action Subsystem1/1(Out1) -> Merge/1
  If Action Subsystem2/1(Out1) -> Merge/2
  Merge/1 -> Out1/1

== system TBCC_Dyn/控制器B/If Action Subsystem1/If Action Subsystem2 ==
  note: 惯性环节
  In1 : Inport
  Action Port : ActionPort  ActionPortLabel=else
  Transfer Fcn (with initial outputs) : simulink_extras/Additional Linear/Transfer Fcn (with initial outputs)  N=[1]  D="[10  1]"  Y0=11000  U0=0
  Out1 : Outport
  wires:
  In1/1 -> Transfer Fcn (with initial outputs)/1
  Transfer Fcn (with initial outputs)/1 -> Out1/1

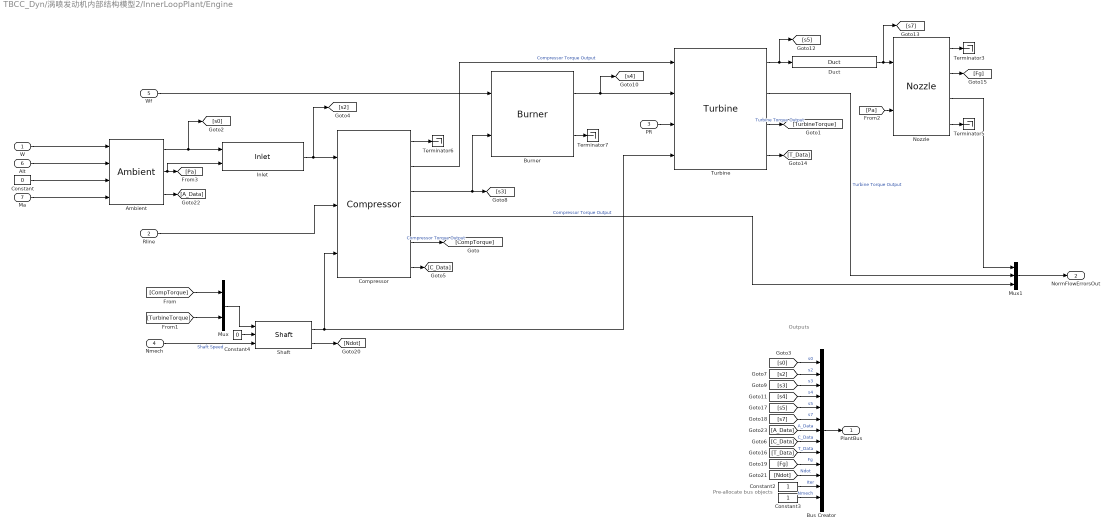
== system TBCC_Dyn/涡喷发动机内部结构模型2/InnerLoopPlant/Engine ==
  note: Pre-allocate bus objects
  note: Outputs
  W : Inport
  Rline : Inport  Port=2
  PR : Inport  Port=3
  Nmech : Inport  Port=4
  Wf : Inport  Port=5
  Alt : Inport  Port=6
  Ma : Inport  Port=7
  Ambient : Lib_Turbo_Ambient_TMATS/Ambient  X_A_AltVec_M=5000*[-1 0 1 2 3 4 5 6 7 8 9 10 12 14 16]  T_A_TsVec_M=[536.51 518.67 500.84 483.03 465.22 447.41 429.62 411.84 394.06 389.97 389.97 389.97 389.97 392.25 397.69]  T_A_PsVec_M=[17.554 14.696 12.228 10.108 8.297 6.759 5.461 4.373 3.468 2.73 2.149 1.692 1.049 0.651 0.406]  AFARc_M=0  X_A_FARVec_M=[0; 0.0050; 0.0100; 0.0150; 0.0200; 0.0250; 0.0300]  T_A_RtArray_M="[0.0686;    0.0686;    0.0686;    0.0686;    0.0686;    0.0686;    0.0686]"  Y_A_TVec_M=[300 10000]  T_A_gammaArray_M=[ 1.4 1.4 1.4 1.4 1.4 1.4 1.4; 1.4 1.4 1.4 1.4 1.4 1.4 1.4]
  Burner : Lib_Turbo_Burner_TMATS/Burner  LHVEn_M=on  LHV_M=MWS.Burner.LHV  Eff_M=1  hFuel_M=-1200  dPnormBurner_M=MWS.Burner.dP
  Bus Creator : BusCreator  Inputs=13
  Compressor : Lib_Turbo_Compressor_TMATS/Compressor  X_C_RlineVec_M=MWS.HPC.RlineVec  Z_C_AlphaVec_M=1  Y_C_Map_NcVec_M=MWS.HPC.NcVec  T_C_Map_WcArray_M=MWS.HPC.WcArray  T_C_Map_PRArray_M=MWS.HPC.PRArray  T_C_Map_EffArray_M=MWS.HPC.EffArray  s_C_Nc_M=MWS.HPC.s_Nc  s_C_Wc_M=MWS.HPC.s_Wc  s_C_PR_M=MWS.HPC.s_PR  s_C_Eff_M=MWS.HPC.s_eff  SL_M=off  Scale_M=none  CBLDEN_M=off  C_CBD_M=0  C_CBFht_M=0.5  C_CBFPt_M=0.5  FBLDEN_M=off  C_FBD_M=0  C_BFht_M=0.5  C_BFPt_M=0.5  DefSMEn_M=off  SMNEn_M=off  SRline_M=1  X_C_Map_WcSurgeVec_M=MWS.HPC.WcMapSurge  T_C_Map_PRSurgeVec_M=MWS.HPC.PRMapSurge  iDesign_M=2  NcDes_M=10000  EffDes_M=0.85  PRDes_M=20  RlineDes_M=2  FVar_M=strcat('iDes_',stripchar_TMATS(gcb),'.bin')  BlkNm_M=double(gcb)  HP_M=off
  Constant : Constant  Value=0
  Constant2 : Constant  OutDataTypeStr=int32
  Constant3 : Constant
  Constant4 : Constant  Value=0
  Duct : Lib_Turbo_Duct_TMATS/Duct  dP_M=MWS.Duct.dP
  Inlet : Lib_Turbo_Inlet_TMATS/Inlet  eRambase_M=MWS.Inlet.eRambase  X_eRamVec_M=[0 3]  T_eRamtbl_M=[1 1]
  Mux : Mux  Inputs=2
  Mux1 : Mux  Inputs=3
  Nozzle : Lib_Turbo_Nozzle_TMATS/Nozzle  SWType_M=Convergent  N_TArea_M=MWS.Noz.ATh  N_EArea_M=110.7  N_FL_M=MWS.Noz.LossPerc  X_N_TtVec2_M=MWS.Noz.TtVec  T_N_TGArray_M=MWS.Noz.TGArray  X_N_PEQPaVec_M=MWS.Noz.PeQPaVec  T_N_CdThArray_M=MWS.Noz.CdThArray  T_N_CvArray_M=MWS.Noz.CvArray  CfgEn_M=off  T_N_CfgArray_M=[1 1]  X_N_FARVec_M=MWS.Noz.FARVec  T_N_RtArray_M=MWS.Noz.RArray  Y_N_TtVec_M=MWS.Noz.TtVec  T_N_MAP_gammaArray_M=MWS.Noz.GArray  iDesign_M=2  WDes_M=100  FVar_M=strcat('iDes_',stripchar_TMATS(gcb),'.bin')
  Shaft : Lib_Turbo_Shaft_TMATS/Shaft  Shaft_Inertia_M=MWS.Shaft.N_I
  Terminator{3,5..7} (4 alike) : Terminator
  Turbine : Lib_Turbo_Turbine_TMATS/Turbine  X_T_Map_PRVec_M=MWS.HPT.PRVec  Y_T_Map_NcVec_M=MWS.HPT.NcVec  T_T_Map_WcArray_M=MWS.HPT.WcArray  T_T_Map_EffArray_M=MWS.HPT.EffArray  s_T_Nc_M=MWS.HPT.s_Nc  s_T_Wc_M=MWS.HPT.s_Wc  s_T_PR_M=MWS.HPT.s_PR  s_T_Eff_M=MWS.HPT.s_eff  ConfigNPSS_M=0  Scale_M=none  CFlwEn_M=off  T_CoolFlwPos_M=0  iDesign_M=2  NcDes_M=100  EffDes_M=0.9200  PRDes_M=5  NDes_M=10000  FVar_M=strcat('iDes_',stripchar_TMATS(gcb),'.bin')  BlkNm_M=double(gcb)  HP_M=off
  PlantBus : Outport
  NormFlowErrorsOut : Outport  Port=2
  wires:
  Compressor/6 -> [C_Data]
  Ambient/1 -> [s0], Inlet/1
  Duct/1 -> [s7], Nozzle/1
  Ambient/3 -> [A_Data]
  Ambient/2 -> [Pa], Inlet/2
  Ma/1 -> Ambient/4
  Constant/1 -> Ambient/3
  W/1 -> Ambient/1
  Nozzle/2 -> [Fg]
  Compressor/2 -> Turbine/1  "Compressor Torque Output"
  Compressor/1 -> Terminator6/1
  Shaft/1 -> Compressor/3, Turbine/4
  [TurbineTorque] -> Mux/2
  [CompTorque] -> Mux/1
  Turbine/3 -> [TurbineTorque]  "Turbine Torque Output"
  Compressor/5 -> [CompTorque]  "Compressor Torque Output"
  Mux/1 -> Shaft/1
  Shaft/2 -> [Ndot]
  Nmech/1 -> Shaft/3  "Shaft Speed"
  Inlet/1 -> [s2], Compressor/1
  Alt/1 -> Ambient/2
  Compressor/4 -> Mux1/3  "Compressor Torque Output"
  Turbine/2 -> Mux1/2  "Turbine Torque Output"
  Nozzle/4 -> Terminator5/1
  Nozzle/3 -> Mux1/1
  Nozzle/1 -> Terminator3/1
  Turbine/4 -> [T_Data]
  Mux1/1 -> NormFlowErrorsOut/1
  Rline/1 -> Compressor/2
  PR/1 -> Turbine/3
  Turbine/1 -> [s5], Duct/1
  Burner/1 -> [s4], Turbine/2
  [Pa] -> Nozzle/2
  Burner/2 -> Terminator7/1
  Wf/1 -> Burner/1
  Compressor/3 -> [s3], Burner/2
  [s0] -> Bus Creator/1  "s0"
  [s2] -> Bus Creator/2  "s2"
  [s3] -> Bus Creator/3  "s3"
  [s4] -> Bus Creator/4  "s4"
  [s5] -> Bus Creator/5  "s5"
  [s7] -> Bus Creator/6  "s7"
  [C_Data] -> Bus Creator/8  "C_Data"
  [T_Data] -> Bus Creator/9  "T_Data"
  [Fg] -> Bus Creator/10  "Fg"
  [Ndot] -> Bus Creator/11  "Ndot"
  Bus Creator/1 -> PlantBus/1
  [A_Data] -> Bus Creator/7  "A_Data"
  Constant2/1 -> Bus Creator/12  "Iter"
  Constant3/1 -> Bus Creator/13  "Nmech"
  Constant4/1 -> Shaft/2

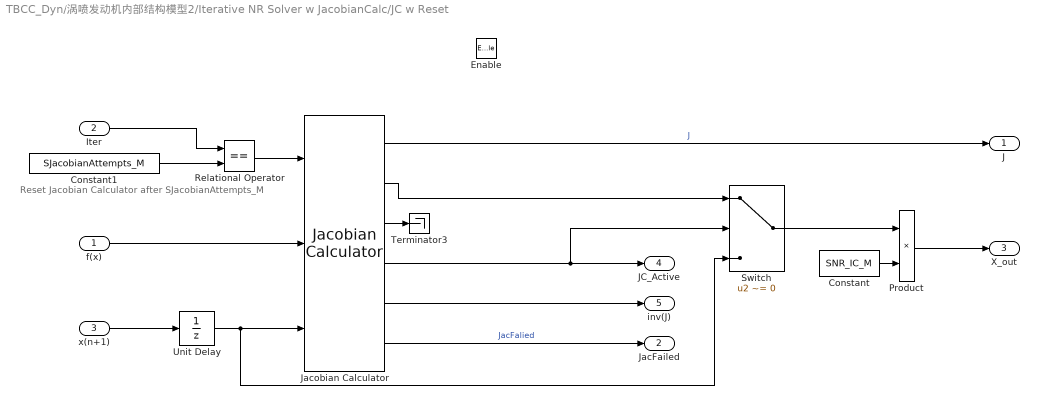
== system TBCC_Dyn/涡喷发动机内部结构模型2/Iterative NR Solver w JacobianCalc/JC w Reset ==
  note: Reset Jacobian Calculator after SJacobianAttempts_M
  f(x) : Inport  PortDimensions=length(SNR_IC_M)
  Iter : Inport  Port=2  PortDimensions=1
  x(n+1) : Inport  Port=3
  Enable : EnablePort
  Constant : Constant  Value=SNR_IC_M
  Constant1 : Constant  Value=SJacobianAttempts_M  OutDataTypeStr=uint32
  Jacobian Calculator : Lib_NM_JacobianCalc_TMATS/Jacobian Calculator  N_Per_M=SJac_Per_M
  Product : Product  RndMeth=Zero
  Relational Operator : RelationalOperator  Operator===  OutDataTypeStr=boolean  RndMeth=Nearest
  Switch : Switch  Criteria=u2 ~= 0  Threshold=1
  Terminator3 : Terminator
  Unit Delay : UnitDelay  InitialCondition=ones(length(SNR_IC_M),1)  SampleTime=-1  HasFrameUpgradeWarning=on
  J : Outport  PortDimensions=[length(SNR_IC_M),length(SNR_IC_M)]
  JacFailed : Outport  Port=2  PortDimensions=1
  X_out : Outport  Port=3  PortDimensions=length(SNR_IC_M)
  JC_Active : Outport  Port=4  PortDimensions=1
  inv(J) : Outport  Port=5  PortDimensions=[length(SNR_IC_M),length(SNR_IC_M)]
  wires:
  Jacobian Calculator/6 -> JacFailed/1  "JacFalied"
  Jacobian Calculator/3 -> Terminator3/1
  Iter/1 -> Relational Operator/1
  Constant1/1 -> Relational Operator/2
  Jacobian Calculator/4 -> JC_Active/1, Switch/2
  Switch/1 -> Product/1
  Jacobian Calculator/2 -> Switch/1
  Product/1 -> X_out/1
  Relational Operator/1 -> Jacobian Calculator/1
  Constant/1 -> Product/2
  Jacobian Calculator/1 -> J/1  "J"
  x(n+1)/1 -> Unit Delay/1
  Unit Delay/1 -> Jacobian Calculator/3, Switch/3
  Jacobian Calculator/5 -> inv(J)/1
  f(x)/1 -> Jacobian Calculator/2

== system TBCC_Dyn/涡喷发动机内部结构模型2/Iterative NR Solver w JacobianCalc/NRwCond ==
  note: Enable NR when conditions are not met
      | and Jacobian Calculator is not active
  f(x) : Inport  PortDimensions=length(SNR_IC_M)
  JC_Active : Inport  Port=2  PortDimensions=1
  inv(f'(x)) : Inport  Port=3  PortDimensions=[length(SNR_IC_M),length(SNR_IC_M)]
  Enable : EnablePort
  Iteration Conditions : Subsystem
  Logical Operator : Logic  Operator=NOT  AllPortsSameDT=off  OutDataTypeStr=boolean
  Logical Operator1 : Logic  AllPortsSameDT=off  OutDataTypeStr=boolean
  Newton Raphson Solver : Lib_NM_NewtonRaphsonSolver_TMATS/Newton Raphson Solver  NR_IC_M=ones(size(SNR_IC_M))  NR_dx_Lim_M=SNR_DX_M  NR_Mx_Lim_M=SNR_Mx_M./SNR_IC_M  NR_Mn_Lim_M=SNR_Mn_M./SNR_IC_M  BlkNm_M=double(gcb)
  Terminator : Terminator
  CCnd : Outport  PortDimensions=1
  x(n+1) : Outport  Port=2  PortDimensions=length(SNR_IC_M)
  wires:
  Iteration Conditions/1(Condition) -> CCnd/1, Logical Operator1/2
  Logical Operator/1 -> Logical Operator1/1
  Logical Operator1/1 -> Newton Raphson Solver/1
  inv(f'(x))/1 -> Newton Raphson Solver/2
  Newton Raphson Solver/1 -> Terminator/1
  Newton Raphson Solver/2 -> x(n+1)/1
  JC_Active/1 -> Logical Operator/1
  f(x)/1 -> Newton Raphson Solver/3, Iteration Conditions/1(f(x))

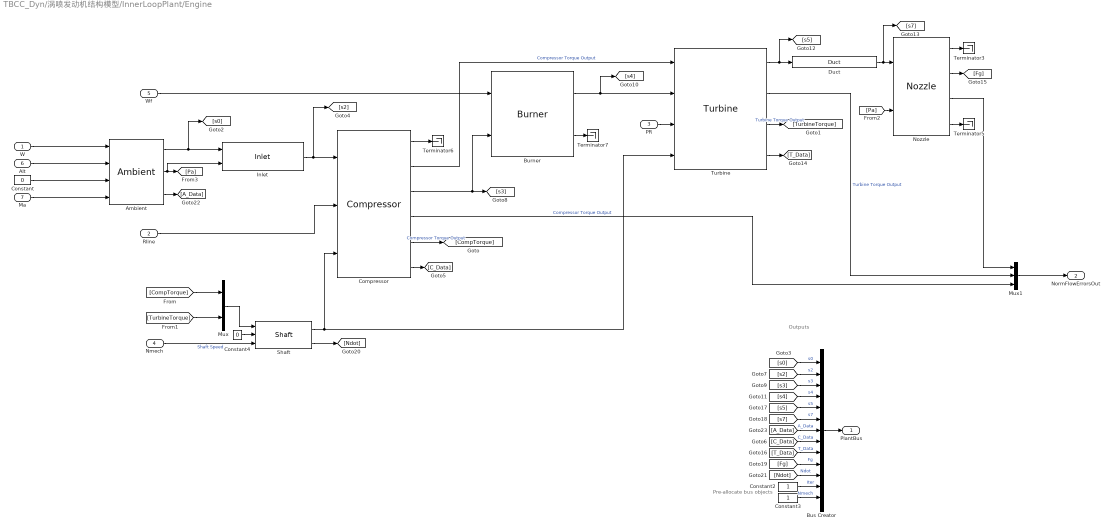
== system TBCC_Dyn/涡喷发动机结构模型/InnerLoopPlant/Engine ==
  note: Pre-allocate bus objects
  note: Outputs
  W : Inport
  Rline : Inport  Port=2
  PR : Inport  Port=3
  Nmech : Inport  Port=4
  Wf : Inport  Port=5
  Alt : Inport  Port=6
  Ma : Inport  Port=7
  Ambient : Lib_Turbo_Ambient_TMATS/Ambient  X_A_AltVec_M=5000*[-1 0 1 2 3 4 5 6 7 8 9 10 12 14 16]  T_A_TsVec_M=[536.51 518.67 500.84 483.03 465.22 447.41 429.62 411.84 394.06 389.97 389.97 389.97 389.97 392.25 397.69]  T_A_PsVec_M=[17.554 14.696 12.228 10.108 8.297 6.759 5.461 4.373 3.468 2.73 2.149 1.692 1.049 0.651 0.406]  AFARc_M=0  X_A_FARVec_M=[0; 0.0050; 0.0100; 0.0150; 0.0200; 0.0250; 0.0300]  T_A_RtArray_M="[0.0686;    0.0686;    0.0686;    0.0686;    0.0686;    0.0686;    0.0686]"  Y_A_TVec_M=[300 10000]  T_A_gammaArray_M=[ 1.4 1.4 1.4 1.4 1.4 1.4 1.4; 1.4 1.4 1.4 1.4 1.4 1.4 1.4]
  Burner : Lib_Turbo_Burner_TMATS/Burner  LHVEn_M=on  LHV_M=MWS.Burner.LHV  Eff_M=1  hFuel_M=-1200  dPnormBurner_M=MWS.Burner.dP
  Bus Creator : BusCreator  Inputs=13
  Compressor : Lib_Turbo_Compressor_TMATS/Compressor  X_C_RlineVec_M=MWS.HPC.RlineVec  Z_C_AlphaVec_M=1  Y_C_Map_NcVec_M=MWS.HPC.NcVec  T_C_Map_WcArray_M=MWS.HPC.WcArray  T_C_Map_PRArray_M=MWS.HPC.PRArray  T_C_Map_EffArray_M=MWS.HPC.EffArray  s_C_Nc_M=MWS.HPC.s_Nc  s_C_Wc_M=MWS.HPC.s_Wc  s_C_PR_M=MWS.HPC.s_PR  s_C_Eff_M=MWS.HPC.s_eff  SL_M=off  Scale_M=none  CBLDEN_M=off  C_CBD_M=0  C_CBFht_M=0.5  C_CBFPt_M=0.5  FBLDEN_M=off  C_FBD_M=0  C_BFht_M=0.5  C_BFPt_M=0.5  DefSMEn_M=off  SMNEn_M=off  SRline_M=1  X_C_Map_WcSurgeVec_M=MWS.HPC.WcMapSurge  T_C_Map_PRSurgeVec_M=MWS.HPC.PRMapSurge  iDesign_M=2  NcDes_M=10000  EffDes_M=0.85  PRDes_M=20  RlineDes_M=2  FVar_M=strcat('iDes_',stripchar_TMATS(gcb),'.bin')  BlkNm_M=double(gcb)  HP_M=off
  Constant : Constant  Value=0
  Constant2 : Constant  OutDataTypeStr=int32
  Constant3 : Constant
  Constant4 : Constant  Value=0
  Duct : Lib_Turbo_Duct_TMATS/Duct  dP_M=MWS.Duct.dP
  Inlet : Lib_Turbo_Inlet_TMATS/Inlet  eRambase_M=MWS.Inlet.eRambase  X_eRamVec_M=[0 3]  T_eRamtbl_M=[1 1]
  Mux : Mux  Inputs=2
  Mux1 : Mux  Inputs=3
  Nozzle : Lib_Turbo_Nozzle_TMATS/Nozzle  SWType_M=Convergent  N_TArea_M=MWS.Noz.ATh  N_EArea_M=110.7  N_FL_M=MWS.Noz.LossPerc  X_N_TtVec2_M=MWS.Noz.TtVec  T_N_TGArray_M=MWS.Noz.TGArray  X_N_PEQPaVec_M=MWS.Noz.PeQPaVec  T_N_CdThArray_M=MWS.Noz.CdThArray  T_N_CvArray_M=MWS.Noz.CvArray  CfgEn_M=off  T_N_CfgArray_M=[1 1]  X_N_FARVec_M=MWS.Noz.FARVec  T_N_RtArray_M=MWS.Noz.RArray  Y_N_TtVec_M=MWS.Noz.TtVec  T_N_MAP_gammaArray_M=MWS.Noz.GArray  iDesign_M=2  WDes_M=100  FVar_M=strcat('iDes_',stripchar_TMATS(gcb),'.bin')
  Shaft : Lib_Turbo_Shaft_TMATS/Shaft  Shaft_Inertia_M=MWS.Shaft.N_I
  Terminator{3,5..7} (4 alike) : Terminator
  Turbine : Lib_Turbo_Turbine_TMATS/Turbine  X_T_Map_PRVec_M=MWS.HPT.PRVec  Y_T_Map_NcVec_M=MWS.HPT.NcVec  T_T_Map_WcArray_M=MWS.HPT.WcArray  T_T_Map_EffArray_M=MWS.HPT.EffArray  s_T_Nc_M=MWS.HPT.s_Nc  s_T_Wc_M=MWS.HPT.s_Wc  s_T_PR_M=MWS.HPT.s_PR  s_T_Eff_M=MWS.HPT.s_eff  ConfigNPSS_M=0  Scale_M=none  CFlwEn_M=off  T_CoolFlwPos_M=0  iDesign_M=2  NcDes_M=100  EffDes_M=0.9200  PRDes_M=5  NDes_M=10000  FVar_M=strcat('iDes_',stripchar_TMATS(gcb),'.bin')  BlkNm_M=double(gcb)  HP_M=off
  PlantBus : Outport
  NormFlowErrorsOut : Outport  Port=2
  wires:
  Compressor/6 -> [C_Data]
  Ambient/1 -> [s0], Inlet/1
  Duct/1 -> [s7], Nozzle/1
  Ambient/3 -> [A_Data]
  Ambient/2 -> [Pa], Inlet/2
  Ma/1 -> Ambient/4
  Constant/1 -> Ambient/3
  W/1 -> Ambient/1
  Nozzle/2 -> [Fg]
  Compressor/2 -> Turbine/1  "Compressor Torque Output"
  Compressor/1 -> Terminator6/1
  Shaft/1 -> Compressor/3, Turbine/4
  [TurbineTorque] -> Mux/2
  [CompTorque] -> Mux/1
  Turbine/3 -> [TurbineTorque]  "Turbine Torque Output"
  Compressor/5 -> [CompTorque]  "Compressor Torque Output"
  Mux/1 -> Shaft/1
  Shaft/2 -> [Ndot]
  Nmech/1 -> Shaft/3  "Shaft Speed"
  Inlet/1 -> [s2], Compressor/1
  Alt/1 -> Ambient/2
  Compressor/4 -> Mux1/3  "Compressor Torque Output"
  Turbine/2 -> Mux1/2  "Turbine Torque Output"
  Nozzle/4 -> Terminator5/1
  Nozzle/3 -> Mux1/1
  Nozzle/1 -> Terminator3/1
  Turbine/4 -> [T_Data]
  Mux1/1 -> NormFlowErrorsOut/1
  Rline/1 -> Compressor/2
  PR/1 -> Turbine/3
  Turbine/1 -> [s5], Duct/1
  Burner/1 -> [s4], Turbine/2
  [Pa] -> Nozzle/2
  Burner/2 -> Terminator7/1
  Wf/1 -> Burner/1
  Compressor/3 -> [s3], Burner/2
  [s0] -> Bus Creator/1  "s0"
  [s2] -> Bus Creator/2  "s2"
  [s3] -> Bus Creator/3  "s3"
  [s4] -> Bus Creator/4  "s4"
  [s5] -> Bus Creator/5  "s5"
  [s7] -> Bus Creator/6  "s7"
  [C_Data] -> Bus Creator/8  "C_Data"
  [T_Data] -> Bus Creator/9  "T_Data"
  [Fg] -> Bus Creator/10  "Fg"
  [Ndot] -> Bus Creator/11  "Ndot"
  Bus Creator/1 -> PlantBus/1
  [A_Data] -> Bus Creator/7  "A_Data"
  Constant2/1 -> Bus Creator/12  "Iter"
  Constant3/1 -> Bus Creator/13  "Nmech"
  Constant4/1 -> Shaft/2

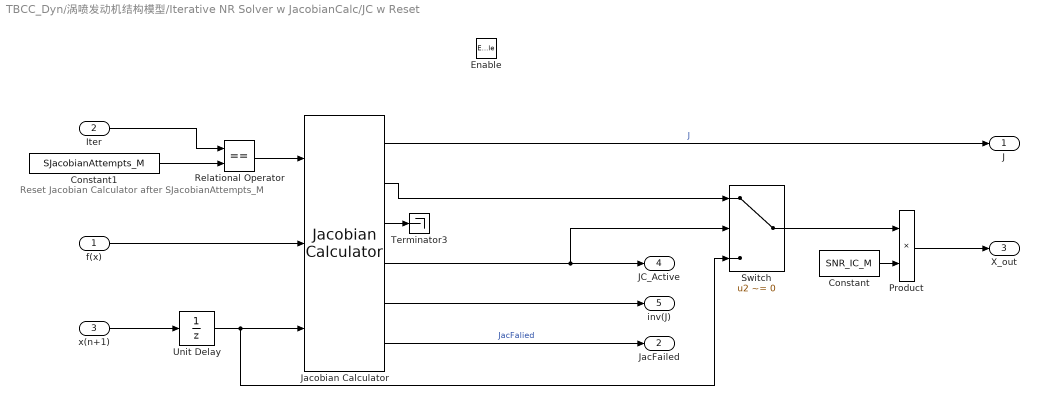
== system TBCC_Dyn/涡喷发动机结构模型/Iterative NR Solver w JacobianCalc/JC w Reset ==
  note: Reset Jacobian Calculator after SJacobianAttempts_M
  f(x) : Inport  PortDimensions=length(SNR_IC_M)
  Iter : Inport  Port=2  PortDimensions=1
  x(n+1) : Inport  Port=3
  Enable : EnablePort
  Constant : Constant  Value=SNR_IC_M
  Constant1 : Constant  Value=SJacobianAttempts_M  OutDataTypeStr=uint32
  Jacobian Calculator : Lib_NM_JacobianCalc_TMATS/Jacobian Calculator  N_Per_M=SJac_Per_M
  Product : Product  RndMeth=Zero
  Relational Operator : RelationalOperator  Operator===  OutDataTypeStr=boolean  RndMeth=Nearest
  Switch : Switch  Criteria=u2 ~= 0  Threshold=1
  Terminator3 : Terminator
  Unit Delay : UnitDelay  InitialCondition=ones(length(SNR_IC_M),1)  SampleTime=-1  HasFrameUpgradeWarning=on
  J : Outport  PortDimensions=[length(SNR_IC_M),length(SNR_IC_M)]
  JacFailed : Outport  Port=2  PortDimensions=1
  X_out : Outport  Port=3  PortDimensions=length(SNR_IC_M)
  JC_Active : Outport  Port=4  PortDimensions=1
  inv(J) : Outport  Port=5  PortDimensions=[length(SNR_IC_M),length(SNR_IC_M)]
  wires:
  Jacobian Calculator/6 -> JacFailed/1  "JacFalied"
  Jacobian Calculator/3 -> Terminator3/1
  Iter/1 -> Relational Operator/1
  Constant1/1 -> Relational Operator/2
  Jacobian Calculator/4 -> JC_Active/1, Switch/2
  Switch/1 -> Product/1
  Jacobian Calculator/2 -> Switch/1
  Product/1 -> X_out/1
  Relational Operator/1 -> Jacobian Calculator/1
  Constant/1 -> Product/2
  Jacobian Calculator/1 -> J/1  "J"
  x(n+1)/1 -> Unit Delay/1
  Unit Delay/1 -> Jacobian Calculator/3, Switch/3
  Jacobian Calculator/5 -> inv(J)/1
  f(x)/1 -> Jacobian Calculator/2
